simulink model "Model_2"  (R2020b)
settings: Solver=VariableStepAuto  StartTime=0.0  StopTime=10.0  RelTol=1e-3
values from neighbouring files (symbols this model uses):
  be = 2    [Variables.m]
  bv = 1    [Variables.m]
  muk = 1    [Variables.m]
  mus = 1.5    [Variables.m]
  R = 1    [Variables.m]
undefined symbols (not defined in the file or in its folder): Ie, Iv
settings Model: Creator=samar  LastModifiedBy=samar

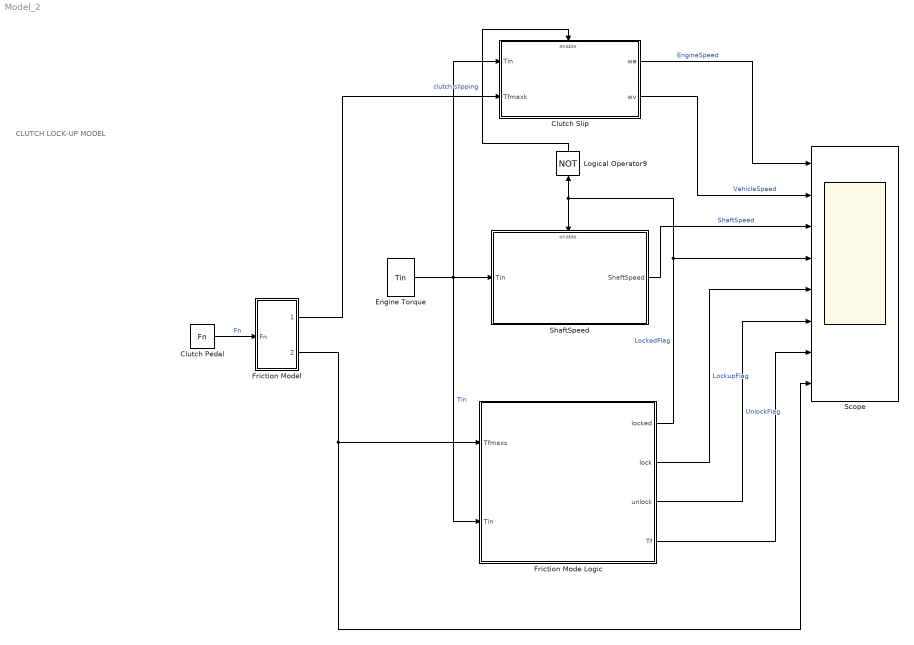
== system Model_2 ==
  note: CLUTCH LOCK-UP MODEL
  Clutch Pedal : FromWorkspace  VariableName=Fn  ZeroCross=off
  Clutch Slip : Subsystem
  Engine Torque : FromWorkspace  VariableName=Tin  ZeroCross=off
  Friction Model : Subsystem
  Friction Mode Logic : Subsystem
  Logical Operator9 : Logic  Operator=NOT  Inputs=1  IconShape=distinctive  OutDataTypeStr=boolean
  Scope : Scope  NumInputPorts=8
  ShaftSpeed : Subsystem
  wires:
  Clutch Pedal/1 -> Friction Model/1(Fn)  "Fn"
  Logical Operator9/1 -> Clutch Slip/Enable  "clutch slipping"
  Friction Model/1(Tfmaxk) -> Clutch Slip/2(Tfmaxk)
  Engine Torque/1 -> Friction Mode Logic/2(Tin), Clutch Slip/1(Tin), ShaftSpeed/1(Tin)  "Tin"
  Friction Model/2(Tfmaxs) -> Scope/8, Friction Mode Logic/1(Tfmaxs)
  Clutch Slip/1(we) -> Scope/1  "EngineSpeed"
  Clutch Slip/2(wv) -> Scope/2  "VehicleSpeed"
  ShaftSpeed/1(ShaftSpeed) -> Scope/3  "ShaftSpeed"
  Friction Mode Logic/1(locked) -> Scope/4, ShaftSpeed/Enable, Logical Operator9/1  "LockedFlag"
  Friction Mode Logic/2(lock) -> Scope/5  "LockupFlag"
  Friction Mode Logic/3(unlock) -> Scope/6  "UnlockFlag"
  Friction Mode Logic/4(Tf) -> Scope/7

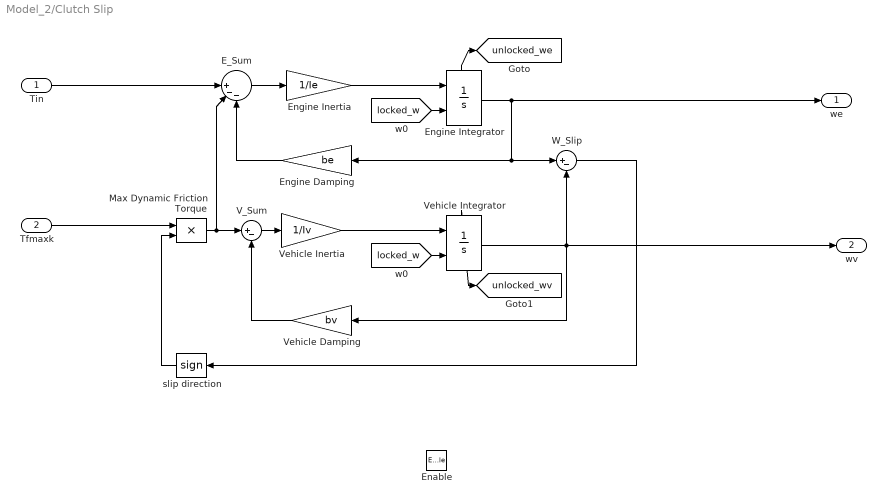
== system Model_2/Clutch Slip ==
  Tin : Inport
  Tfmaxk : Inport  Port=2
  Enable : EnablePort  StatesWhenEnabling=reset
  E_Sum : Sum  Inputs=||+--  InputSameDT=on  SaturateOnIntegerOverflow=on  OutDataTypeStr=Inherit: Same as first input
  Engine Damping : Gain  Gain=be  SaturateOnIntegerOverflow=on  OutDataTypeStr=Inherit: Same as input  ParamDataTypeStr=Inherit: Same as input
  Engine Inertia : Gain  Gain=1/Ie  SaturateOnIntegerOverflow=on  OutDataTypeStr=Inherit: Same as input  ParamDataTypeStr=Inherit: Same as input
  Engine Integrator : Integrator  InitialConditionSource=external  ShowStatePort=on
  Max Dynamic Friction Torque : Product  InputSameDT=on  RndMeth=Zero  SaturateOnIntegerOverflow=on  OutDataTypeStr=Inherit: Same as first input
  V_Sum : Sum  Inputs=|+-  InputSameDT=on  SaturateOnIntegerOverflow=on  OutDataTypeStr=Inherit: Same as first input
  Vehicle Damping : Gain  Gain=bv  SaturateOnIntegerOverflow=on  OutDataTypeStr=Inherit: Same as input  ParamDataTypeStr=Inherit: Same as input
  Vehicle Inertia : Gain  Gain=1/Iv  SaturateOnIntegerOverflow=on  OutDataTypeStr=Inherit: Same as input  ParamDataTypeStr=Inherit: Same as input
  Vehicle Integrator : Integrator  InitialConditionSource=external  ShowStatePort=on
  W_Slip : Sum  Inputs=|+-  InputSameDT=on  SaturateOnIntegerOverflow=on  OutDataTypeStr=Inherit: Same as first input
  slip direction : Signum
  we : Outport
  wv : Outport  Port=2
  tag scope: unlocked_we=global, unlocked_wv=global
  wires:
  Vehicle Integrator/1 -> wv/1, W_Slip/2, Vehicle Damping/1
  [locked_w] -> Vehicle Integrator/2
  V_Sum/1 -> Vehicle Inertia/1
  Vehicle Inertia/1 -> Vehicle Integrator/1
  slip direction/1 -> Max Dynamic Friction Torque/2
  Vehicle Integrator/State -> [unlocked_wv]
  Engine Integrator/1 -> we/1, W_Slip/1, Engine Damping/1
  Engine Damping/1 -> E_Sum/3
  [locked_w] -> Engine Integrator/2
  Vehicle Damping/1 -> V_Sum/2
  W_Slip/1 -> slip direction/1
  Engine Integrator/State -> [unlocked_we]
  E_Sum/1 -> Engine Inertia/1
  Engine Inertia/1 -> Engine Integrator/1
  Max Dynamic Friction Torque/1 -> E_Sum/2, V_Sum/1
  Tin/1 -> E_Sum/1
  Tfmaxk/1 -> Max Dynamic Friction Torque/1

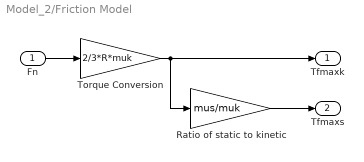
== system Model_2/Friction Model ==
  Fn : Inport
  Ratio of static to kinetic : Gain  Gain=mus/muk  SaturateOnIntegerOverflow=on  OutDataTypeStr=Inherit: Same as input  ParamDataTypeStr=Inherit: Same as input
  Torque Conversion : Gain  Gain=2/3*R*muk  SaturateOnIntegerOverflow=on  OutDataTypeStr=Inherit: Same as input  ParamDataTypeStr=Inherit: Same as input
  Tfmaxk : Outport  InitialOutput=0  VectorParamsAs1DForOutWhenUnconnected=off
  Tfmaxs : Outport  Port=2  InitialOutput=0  VectorParamsAs1DForOutWhenUnconnected=off
  wires:
  Ratio of static to kinetic/1 -> Tfmaxs/1
  Fn/1 -> Torque Conversion/1
  Torque Conversion/1 -> Ratio of static to kinetic/1, Tfmaxk/1

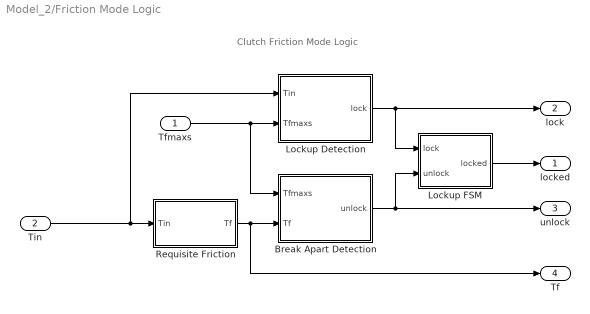
== system Model_2/Friction Mode Logic ==
  note: Clutch Friction Mode Logic
  Tfmaxs : Inport
  Tin : Inport  Port=2
  Break Apart Detection : Subsystem
  Lockup Detection : Subsystem
  Lockup FSM : Subsystem
  Requisite Friction : Subsystem
  locked : Outport
  lock : Outport  Port=2
  unlock : Outport  Port=3
  Tf : Outport  Port=4
  wires:
  Requisite Friction/1(Tf) -> Tf/1, Break Apart Detection/2(Tf)
  Lockup Detection/1(lock) -> lock/1, Lockup FSM/1(lock)
  Tin/1 -> Requisite Friction/1(Tin), Lockup Detection/1(Tin)
  Lockup FSM/1(locked) -> locked/1
  Break Apart Detection/1(unlock) -> unlock/1, Lockup FSM/2(unlock)
  Tfmaxs/1 -> Break Apart Detection/1(Tfmaxs), Lockup Detection/2(Tfmaxs)

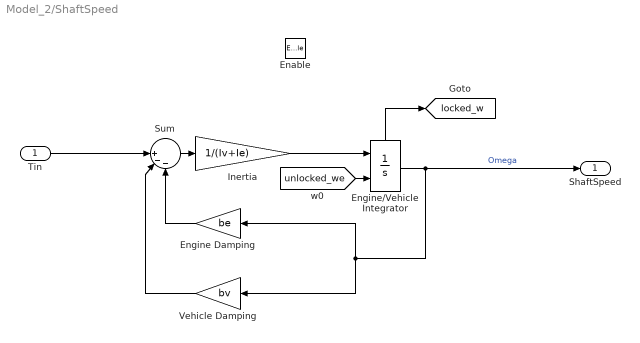
== system Model_2/ShaftSpeed ==
  Tin : Inport
  Enable : EnablePort  StatesWhenEnabling=reset
  Engine Damping : Gain  Gain=be  SaturateOnIntegerOverflow=on  OutDataTypeStr=Inherit: Same as input  ParamDataTypeStr=Inherit: Same as input
  Engine/Vehicle Integrator : Integrator  InitialConditionSource=external  ShowStatePort=on
  Inertia : Gain  Gain=1/(Iv+Ie)  SaturateOnIntegerOverflow=on  OutDataTypeStr=Inherit: Same as input  ParamDataTypeStr=Inherit: Same as input
  Sum : Sum  Inputs=||+--  InputSameDT=on  SaturateOnIntegerOverflow=on  OutDataTypeStr=Inherit: Same as first input
  Vehicle Damping : Gain  Gain=bv  SaturateOnIntegerOverflow=on  OutDataTypeStr=Inherit: Same as input  ParamDataTypeStr=Inherit: Same as input
  ShaftSpeed : Outport
  tag scope: locked_w=global
  wires:
  Tin/1 -> Sum/1
  Inertia/1 -> Engine/Vehicle Integrator/1
  Sum/1 -> Inertia/1
  [unlocked_we] -> Engine/Vehicle Integrator/2
  Engine Damping/1 -> Sum/3
  Engine/Vehicle Integrator/1 -> ShaftSpeed/1, Vehicle Damping/1, Engine Damping/1  "Omega"
  Engine/Vehicle Integrator/State -> [locked_w]
  Vehicle Damping/1 -> Sum/2

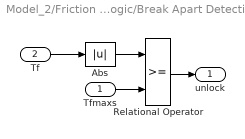
== system Model_2/Friction Mode Logic/Break Apart Detection ==
  Tfmaxs : Inport
  Tf : Inport  Port=2
  Abs : Abs  SaturateOnIntegerOverflow=on
  Relational Operator : RelationalOperator  OutDataTypeStr=boolean  RndMeth=Nearest  InputSameDT=on
  unlock : Outport  InitialOutput=0  VectorParamsAs1DForOutWhenUnconnected=off
  wires:
  Tfmaxs/1 -> Relational Operator/2
  Abs/1 -> Relational Operator/1
  Relational Operator/1 -> unlock/1
  Tf/1 -> Abs/1

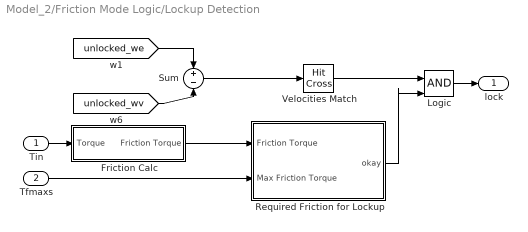
== system Model_2/Friction Mode Logic/Lockup Detection ==
  Tin : Inport
  Tfmaxs : Inport  Port=2
  Friction Calc : Subsystem
  Logic : Logic  IconShape=distinctive  OutDataTypeStr=boolean
  Required Friction for Lockup : Subsystem
  Sum : Sum  Inputs=+-  InputSameDT=on  SaturateOnIntegerOverflow=on  OutDataTypeStr=Inherit: Same as first input
  Velocities Match : HitCross
  lock : Outport  InitialOutput=0  VectorParamsAs1DForOutWhenUnconnected=off
  wires:
  Tin/1 -> Friction Calc/1(Torque)
  Sum/1 -> Velocities Match/1
  [unlocked_wv] -> Sum/2
  [unlocked_we] -> Sum/1
  Required Friction for Lockup/1(okay) -> Logic/2
  Logic/1 -> lock/1
  Velocities Match/1 -> Logic/1
  Tfmaxs/1 -> Required Friction for Lockup/2(Max Friction Torque)
  Friction Calc/1(Friction Torque) -> Required Friction for Lockup/1(Friction Torque)

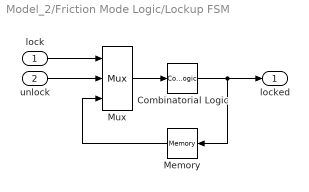
== system Model_2/Friction Mode Logic/Lockup FSM ==
  lock : Inport
  unlock : Inport  Port=2
  Combinatorial Logic : CombinatorialLogic  TruthTable=[0;1;0;0;1;1;1;0]
  Memory : Memory
  Mux : Mux  Inputs=3
  locked : Outport  InitialOutput=0  VectorParamsAs1DForOutWhenUnconnected=off
  wires:
  Mux/1 -> Combinatorial Logic/1
  lock/1 -> Mux/1
  unlock/1 -> Mux/2
  Combinatorial Logic/1 -> Memory/1, locked/1
  Memory/1 -> Mux/3

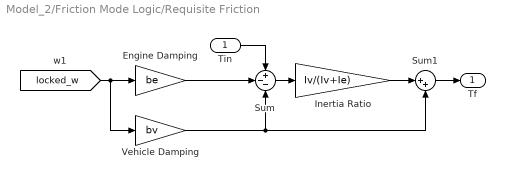
== system Model_2/Friction Mode Logic/Requisite Friction ==
  Tin : Inport
  Engine Damping : Gain  Gain=be  SaturateOnIntegerOverflow=on  OutDataTypeStr=Inherit: Same as input  ParamDataTypeStr=Inherit: Same as input
  Inertia Ratio : Gain  Gain=Iv/(Iv+Ie)  SaturateOnIntegerOverflow=on  OutDataTypeStr=Inherit: Same as input  ParamDataTypeStr=Inherit: Same as input
  Sum : Sum  Inputs=+--  InputSameDT=on  SaturateOnIntegerOverflow=on  OutDataTypeStr=Inherit: Same as first input
  Sum1 : Sum  Inputs=|++  InputSameDT=on  SaturateOnIntegerOverflow=on  OutDataTypeStr=Inherit: Same as first input
  Vehicle Damping : Gain  Gain=bv  SaturateOnIntegerOverflow=on  OutDataTypeStr=Inherit: Same as input  ParamDataTypeStr=Inherit: Same as input
  Tf : Outport  InitialOutput=0  VectorParamsAs1DForOutWhenUnconnected=off
  wires:
  Sum1/1 -> Tf/1
  Inertia Ratio/1 -> Sum1/1
  Tin/1 -> Sum/1
  Sum/1 -> Inertia Ratio/1
  Vehicle Damping/1 -> Sum1/2, Sum/3
  Engine Damping/1 -> Sum/2
  [locked_w] -> Engine Damping/1, Vehicle Damping/1

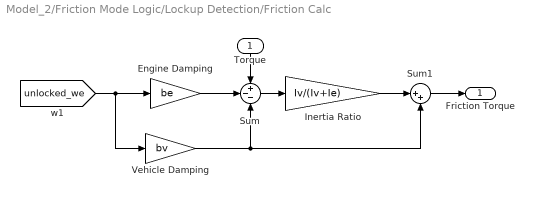
== system Model_2/Friction Mode Logic/Lockup Detection/Friction Calc ==
  Torque : Inport
  Engine Damping : Gain  Gain=be  SaturateOnIntegerOverflow=on  OutDataTypeStr=Inherit: Same as input  ParamDataTypeStr=Inherit: Same as input
  Inertia Ratio : Gain  Gain=Iv/(Iv+Ie)  SaturateOnIntegerOverflow=on  OutDataTypeStr=Inherit: Same as input  ParamDataTypeStr=Inherit: Same as input
  Sum : Sum  Inputs=+--  InputSameDT=on  SaturateOnIntegerOverflow=on  OutDataTypeStr=Inherit: Same as first input
  Sum1 : Sum  Inputs=|++  InputSameDT=on  SaturateOnIntegerOverflow=on  OutDataTypeStr=Inherit: Same as first input
  Vehicle Damping : Gain  Gain=bv  SaturateOnIntegerOverflow=on  OutDataTypeStr=Inherit: Same as input  ParamDataTypeStr=Inherit: Same as input
  Friction Torque : Outport  InitialOutput=0  VectorParamsAs1DForOutWhenUnconnected=off
  wires:
  Sum1/1 -> Friction Torque/1
  Inertia Ratio/1 -> Sum1/1
  Torque/1 -> Sum/1
  Sum/1 -> Inertia Ratio/1
  Engine Damping/1 -> Sum/2
  Vehicle Damping/1 -> Sum/3, Sum1/2
  [unlocked_we] -> Vehicle Damping/1, Engine Damping/1

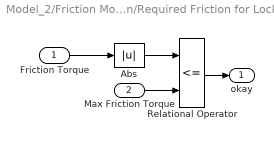
== system Model_2/Friction Mode Logic/Lockup Detection/Required Friction for Lockup ==
  Friction Torque : Inport
  Max Friction Torque : Inport  Port=2
  Abs : Abs  SaturateOnIntegerOverflow=on
  Relational Operator : RelationalOperator  Operator=<=  OutDataTypeStr=boolean  RndMeth=Nearest  InputSameDT=on
  okay : Outport  InitialOutput=0  VectorParamsAs1DForOutWhenUnconnected=off
  wires:
  Max Friction Torque/1 -> Relational Operator/2
  Abs/1 -> Relational Operator/1
  Relational Operator/1 -> okay/1
  Friction Torque/1 -> Abs/1
